simulink model "APP_MyApplication"  (R2018b)
settings: Solver=VariableStepDiscrete  StartTime=0.0  StopTime=10  RelTol=1e-3
PreLoadFcn:
  | if(exist('MBDS_ModelCallback', 'file')), MBDS_ModelCallback('PreLoad'); end;
PostLoadFcn:
  | if(exist('MBDS_ModelCallback', 'file')), MBDS_ModelCallback('PostLoad'); end;
InitFcn:
  | if(exist('MBDS_ModelCallback', 'file')), MBDS_ModelCallback('Init'); end;
StartFcn:
  | if(exist('MBDS_ModelCallback', 'file')), MBDS_ModelCallback('Start'); end;
StopFcn:
  | if(exist('MBDS_ModelCallback', 'file')), MBDS_ModelCallback('Stop'); end;
undefined symbols (not defined in the file): sigbuilder_block, Ts
libraries: KIBES_Signal x499, simulink x8
(part 5 of 10)

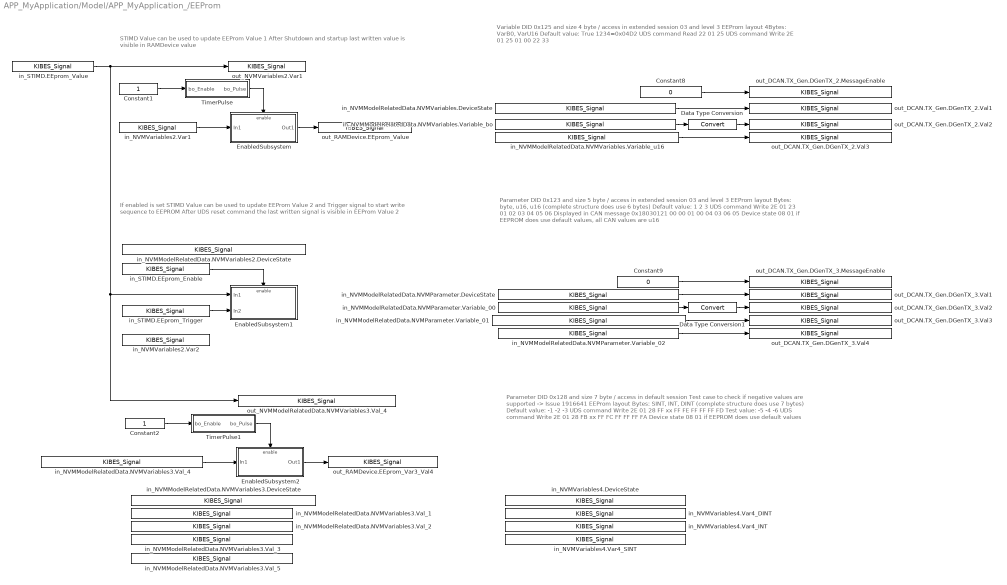
== system APP_MyApplication/Model/APP_MyApplication_/EEProm ==
  note: STIMD Value can be used to update EEProm Value 1
      | After Shutdown and startup last written value is visible in RAMDevice value
  note: Parameter DID 0x123 and size 5 byte / access in extended session 03 and level 3
      | EEProm layout Bytes: byte, u16, u16 (complete structure does use 6 bytes)
      | Default value: 1 2 3
      | UDS command Write 2E 01 23 01 02 03 04 05 06
      | Displayed in CAN message 0x18030121 00 00 01 00 04 03 06 05
      | Device state 08 01 if EEPROM does use default values, all CAN values are u16
  note: Variable DID 0x125 and size 4 byte / access in extended session 03 and level 3
      | EEProm layout 4Bytes: VarB0, VarU16
      | Default value: True 1234=0x04D2
      | UDS command Read 22 01 25
      | UDS command Write 2E 01 25 01 00 22 33
  note: If enabled is set
      | STIMD Value can be used to update EEProm Value 2
      | and Trigger signal to start write sequence to EEPROM
      | After UDS reset command the last written signal is visible in EEProm Value 2
  note: Parameter DID 0x128 and size 7 byte / access in default session
      | Test case to check if negative values are supported -> Issue 1916641
      | EEProm layout Bytes: SINT, INT, DINT (complete structure does use 7 bytes)
      | Default value: -1 -2 -3
      | UDS command Write 2E 01 28 FF xx FF FE FF FF FF FD
      | Test value: -5 -4 -6
      | UDS command Write 2E 01 28 FB xx FF FC FF FF FF FA
      | Device state 08 01 if EEPROM does use default values
  Constant1 : Constant  InitFcn=|  OutDataTypeStr=boolean
      | if(exist('MBDS_BlockCallback', 'file'))
      |    MBDS_BlockCallback('Update', gcb);  
      | end
  Constant2 : Constant  InitFcn=|  OutDataTypeStr=boolean
      | if(exist('MBDS_BlockCallback', 'file'))
      |    MBDS_BlockCallback('Update', gcb);  
      | end
  Constant8 : Constant  InitFcn=|  Value=0  OutDataTypeStr=boolean
      | if(exist('MBDS_BlockCallback', 'file'))
      |    MBDS_BlockCallback('Update', gcb);  
      | end
  Constant9 : Constant  InitFcn=|  Value=0  OutDataTypeStr=boolean
      | if(exist('MBDS_BlockCallback', 'file'))
      |    MBDS_BlockCallback('Update', gcb);  
      | end
  Data Type Conversion : DataTypeConversion  InitFcn=|  SaturateOnIntegerOverflow=on
      | try
      |    MBDS_BlockCallback('Update', gcb);
      | end
      settings: AttributesFormatString=Saturate: %<SaturateOnIntegerOverflow>
  Data Type Conversion1 : DataTypeConversion  InitFcn=|  SaturateOnIntegerOverflow=on
      | try
      |    MBDS_BlockCallback('Update', gcb);
      | end
      settings: AttributesFormatString=Saturate: %<SaturateOnIntegerOverflow>
  EnabledSubsystem : Subsystem
  EnabledSubsystem1 : Subsystem
  EnabledSubsystem2 : Subsystem
  TimerPulse : Subsystem
  TimerPulse1 : Subsystem
  in_NVMModelRelatedData.NVMParameter.DeviceState : KIBES_Signal/KIBES_Signal  MBDS_LibraryBlock=on  DatabaseKey=167  SignalName=NVMModelRelatedData.NVMParameter.DeviceState  SymbolName=NVMModelRelatedData_NVMParameter_DeviceState_000167  DataType=uint16  Init=0  Slope=1  Bias=0  DataSize=1  fpDataType=uint16  BlockIOType=Inport  DeviceType=0
  in_NVMModelRelatedData.NVMParameter.Variable_00 : KIBES_Signal/KIBES_Signal  MBDS_LibraryBlock=on  DatabaseKey=168  SignalName=NVMModelRelatedData.NVMParameter.Variable_00  SymbolName=NVMModelRelatedData_NVMParameter_Variable_00_000168  DataType=uint8  Init=1  Slope=1  Bias=0  DataSize=1  fpDataType=uint8  BlockIOType=Inport  DeviceType=0
  in_NVMModelRelatedData.NVMParameter.Variable_01 : KIBES_Signal/KIBES_Signal  MBDS_LibraryBlock=on  DatabaseKey=169  SignalName=NVMModelRelatedData.NVMParameter.Variable_01  SymbolName=NVMModelRelatedData_NVMParameter_Variable_01_000169  DataType=uint16  Init=0  Slope=1  Bias=0  DataSize=1  fpDataType=uint16  BlockIOType=Inport  DeviceType=0
  in_NVMModelRelatedData.NVMParameter.Variable_02 : KIBES_Signal/KIBES_Signal  MBDS_LibraryBlock=on  DatabaseKey=170  SignalName=NVMModelRelatedData.NVMParameter.Variable_02  SymbolName=NVMModelRelatedData_NVMParameter_Variable_02_000170  DataType=uint16  Init=3  Slope=1  Bias=0  DataSize=1  fpDataType=uint16  BlockIOType=Inport  DeviceType=0
  in_NVMModelRelatedData.NVMVariables.DeviceState : KIBES_Signal/KIBES_Signal  MBDS_LibraryBlock=on  DatabaseKey=160  SignalName=NVMModelRelatedData.NVMVariables.DeviceState  SymbolName=NVMModelRelatedData_NVMVariables_DeviceState_000160  DataType=uint16  Init=0  Slope=1  Bias=0  DataSize=1  fpDataType=uint16  BlockIOType=Inport  DeviceType=0
  in_NVMModelRelatedData.NVMVariables.Variable_bo : KIBES_Signal/KIBES_Signal  MBDS_LibraryBlock=on  DatabaseKey=161  SignalName=NVMModelRelatedData.NVMVariables.Variable_bo  SymbolName=NVMModelRelatedData_NVMVariables_Variable_bo_000161  DataType=boolean  Init=1  Slope=1  Bias=0  DataSize=1  fpDataType=boolean  BlockIOType=Inport  DeviceType=0
  in_NVMModelRelatedData.NVMVariables.Variable_u16 : KIBES_Signal/KIBES_Signal  MBDS_LibraryBlock=on  DatabaseKey=162  SignalName=NVMModelRelatedData.NVMVariables.Variable_u16  SymbolName=NVMModelRelatedData_NVMVariables_Variable_u16_000162  DataType=uint16  Init=1234  Slope=1  Bias=0  DataSize=1  fpDataType=uint16  BlockIOType=Inport  DeviceType=0
  in_NVMModelRelatedData.NVMVariables2.DeviceState : KIBES_Signal/KIBES_Signal  MBDS_LibraryBlock=on  DatabaseKey=439  SignalName=NVMModelRelatedData.NVMVariables2.DeviceState  SymbolName=NVMModelRelatedData_NVMVariables2_DeviceState_000439  DataType=uint16  Init=0  Slope=1  Bias=0  DataSize=1  fpDataType=uint16  BlockIOType=Inport  DeviceType=0
  in_NVMModelRelatedData.NVMVariables3.DeviceState : KIBES_Signal/KIBES_Signal  MBDS_LibraryBlock=on  DatabaseKey=536  SignalName=NVMModelRelatedData.NVMVariables3.DeviceState  SymbolName=NVMModelRelatedData_NVMVariables3_DeviceState_000536  DataType=uint16  Init=0  Slope=1  Bias=0  DataSize=1  fpDataType=uint16  BlockIOType=Inport  DeviceType=0
  in_NVMModelRelatedData.NVMVariables3.Val_1 : KIBES_Signal/KIBES_Signal  MBDS_LibraryBlock=on  DatabaseKey=537  SignalName=NVMModelRelatedData.NVMVariables3.Val_1  SymbolName=NVMModelRelatedData_NVMVariables3_Val_1_000537  DataType=boolean  Init=1  Slope=1  Bias=0  DataSize=1  fpDataType=boolean  BlockIOType=Inport  DeviceType=0
  in_NVMModelRelatedData.NVMVariables3.Val_2 : KIBES_Signal/KIBES_Signal  MBDS_LibraryBlock=on  DatabaseKey=538  SignalName=NVMModelRelatedData.NVMVariables3.Val_2  SymbolName=NVMModelRelatedData_NVMVariables3_Val_2_000538  DataType=uint8  Init=2  Slope=1  Bias=0  DataSize=1  fpDataType=uint8  BlockIOType=Inport  DeviceType=0
  in_NVMModelRelatedData.NVMVariables3.Val_3 : KIBES_Signal/KIBES_Signal  MBDS_LibraryBlock=on  DatabaseKey=539  SignalName=NVMModelRelatedData.NVMVariables3.Val_3  SymbolName=NVMModelRelatedData_NVMVariables3_Val_3_000539  DataType=uint16  Init=3  Slope=1  Bias=0  DataSize=1  fpDataType=uint16  BlockIOType=Inport  DeviceType=0
  in_NVMModelRelatedData.NVMVariables3.Val_4 : KIBES_Signal/KIBES_Signal  MBDS_LibraryBlock=on  DatabaseKey=540  SignalName=NVMModelRelatedData.NVMVariables3.Val_4  SymbolName=NVMModelRelatedData_NVMVariables3_Val_4_000540  DataType=uint32  Init=4  Slope=1  Bias=0  DataSize=1  fpDataType=uint32  BlockIOType=Inport  DeviceType=0
  in_NVMModelRelatedData.NVMVariables3.Val_5 : KIBES_Signal/KIBES_Signal  MBDS_LibraryBlock=on  DatabaseKey=542  SignalName=NVMModelRelatedData.NVMVariables3.Val_5  SymbolName=NVMModelRelatedData_NVMVariables3_Val_5_000542  DataType=uint8  Init=0  Slope=1  Bias=0  DataSize=1  fpDataType=uint8  BlockIOType=Inport  DeviceType=0
  in_NVMVariables2.Var1 : KIBES_Signal/KIBES_Signal  MBDS_LibraryBlock=on  DatabaseKey=438  SignalName=NVMVariables2.Var1  SymbolName=NVMVariables2_Var1_000438  DataType=uint32  Init=0  Slope=1  Bias=0  DataSize=1  fpDataType=uint32  BlockIOType=Inport  DeviceType=0
  in_NVMVariables2.Var2 : KIBES_Signal/KIBES_Signal  MBDS_LibraryBlock=on  DatabaseKey=437  SignalName=NVMVariables2.Var2  SymbolName=NVMVariables2_Var2_000437  DataType=uint32  Init=0  Slope=1  Bias=0  DataSize=1  fpDataType=uint32  BlockIOType=Inport  DeviceType=0
  in_NVMVariables4.DeviceState : KIBES_Signal/KIBES_Signal  MBDS_LibraryBlock=on  DatabaseKey=607  SignalName=NVMVariables4.DeviceState  SymbolName=NVMVariables4_DeviceState_000607  DataType=uint16  Init=0  Slope=1  Bias=0  DataSize=1  fpDataType=uint16  BlockIOType=Inport  DeviceType=0
  in_NVMVariables4.Var4_DINT : KIBES_Signal/KIBES_Signal  MBDS_LibraryBlock=on  DatabaseKey=605  SignalName=NVMVariables4.Var4_DINT  SymbolName=NVMVariables4_Var4_DINT_000605  DataType=int32  Init=0  Slope=1  Bias=0  DataSize=1  fpDataType=int32  BlockIOType=Inport  DeviceType=0
  in_NVMVariables4.Var4_INT : KIBES_Signal/KIBES_Signal  MBDS_LibraryBlock=on  DatabaseKey=604  SignalName=NVMVariables4.Var4_INT  SymbolName=NVMVariables4_Var4_INT_000604  DataType=int16  Init=0  Slope=1  Bias=0  DataSize=1  fpDataType=int16  BlockIOType=Inport  DeviceType=0
  in_NVMVariables4.Var4_SINT : KIBES_Signal/KIBES_Signal  MBDS_LibraryBlock=on  DatabaseKey=606  SignalName=NVMVariables4.Var4_SINT  SymbolName=NVMVariables4_Var4_SINT_000606  DataType=int8  Init=0  Slope=1  Bias=0  DataSize=1  fpDataType=int8  BlockIOType=Inport  DeviceType=0
  in_STIMD.EEprom_Enable : KIBES_Signal/KIBES_Signal  MBDS_LibraryBlock=on  DatabaseKey=433  SignalName=STIMD.EEprom_Enable  SymbolName=STIMD_EEprom_Enable_000433  DataType=boolean  Init=0  Slope=1  Bias=0  DataSize=1  fpDataType=boolean  BlockIOType=Inport  DeviceType=2
  in_STIMD.EEprom_Trigger : KIBES_Signal/KIBES_Signal  MBDS_LibraryBlock=on  DatabaseKey=434  SignalName=STIMD.EEprom_Trigger  SymbolName=STIMD_EEprom_Trigger_000434  DataType=boolean  Init=0  Slope=1  Bias=0  DataSize=1  fpDataType=boolean  BlockIOType=Inport  DeviceType=2
  in_STIMD.EEprom_Value : KIBES_Signal/KIBES_Signal  MBDS_LibraryBlock=on  DatabaseKey=435  SignalName=STIMD.EEprom_Value  SymbolName=STIMD_EEprom_Value_000435  DataType=uint32  Init=0  Slope=1  Bias=0  DataSize=1  fpDataType=uint32  BlockIOType=Inport  DeviceType=2
  out_DCAN.TX_Gen.DGenTX_2.MessageEnable : KIBES_Signal/KIBES_Signal  MBDS_LibraryBlock=on  DatabaseKey=163  SignalName=DCAN.TX_Gen.DGenTX_2.MessageEnable  SymbolName=DCAN_TX_Gen_DGenTX_2_MessageEnable_000163  DataType=boolean  Init=0  Slope=1  Bias=0  DataSize=1  fpDataType=boolean  BlockIOType=Outport  DeviceType=0
  out_DCAN.TX_Gen.DGenTX_2.Val1 : KIBES_Signal/KIBES_Signal  MBDS_LibraryBlock=on  DatabaseKey=164  SignalName=DCAN.TX_Gen.DGenTX_2.Val1  SymbolName=DCAN_TX_Gen_DGenTX_2_Val1_000164  DataType=uint16  Init=0  Slope=1  Bias=0  DataSize=1  fpDataType=uint16  BlockIOType=Outport  DeviceType=0
  out_DCAN.TX_Gen.DGenTX_2.Val2 : KIBES_Signal/KIBES_Signal  MBDS_LibraryBlock=on  DatabaseKey=165  SignalName=DCAN.TX_Gen.DGenTX_2.Val2  SymbolName=DCAN_TX_Gen_DGenTX_2_Val2_000165  DataType=uint16  Init=0  Slope=1  Bias=0  DataSize=1  fpDataType=uint16  BlockIOType=Outport  DeviceType=0
  out_DCAN.TX_Gen.DGenTX_2.Val3 : KIBES_Signal/KIBES_Signal  MBDS_LibraryBlock=on  DatabaseKey=166  SignalName=DCAN.TX_Gen.DGenTX_2.Val3  SymbolName=DCAN_TX_Gen_DGenTX_2_Val3_000166  DataType=uint16  Init=0  Slope=1  Bias=0  DataSize=1  fpDataType=uint16  BlockIOType=Outport  DeviceType=0
  out_DCAN.TX_Gen.DGenTX_3.MessageEnable : KIBES_Signal/KIBES_Signal  MBDS_LibraryBlock=on  DatabaseKey=171  SignalName=DCAN.TX_Gen.DGenTX_3.MessageEnable  SymbolName=DCAN_TX_Gen_DGenTX_3_MessageEnable_000171  DataType=boolean  Init=0  Slope=1  Bias=0  DataSize=1  fpDataType=boolean  BlockIOType=Outport  DeviceType=0
  out_DCAN.TX_Gen.DGenTX_3.Val1 : KIBES_Signal/KIBES_Signal  MBDS_LibraryBlock=on  DatabaseKey=172  SignalName=DCAN.TX_Gen.DGenTX_3.Val1  SymbolName=DCAN_TX_Gen_DGenTX_3_Val1_000172  DataType=uint16  Init=0  Slope=1  Bias=0  DataSize=1  fpDataType=uint16  BlockIOType=Outport  DeviceType=0
  out_DCAN.TX_Gen.DGenTX_3.Val2 : KIBES_Signal/KIBES_Signal  MBDS_LibraryBlock=on  DatabaseKey=173  SignalName=DCAN.TX_Gen.DGenTX_3.Val2  SymbolName=DCAN_TX_Gen_DGenTX_3_Val2_000173  DataType=uint16  Init=0  Slope=1  Bias=0  DataSize=1  fpDataType=uint16  BlockIOType=Outport  DeviceType=0
  out_DCAN.TX_Gen.DGenTX_3.Val3 : KIBES_Signal/KIBES_Signal  MBDS_LibraryBlock=on  DatabaseKey=174  SignalName=DCAN.TX_Gen.DGenTX_3.Val3  SymbolName=DCAN_TX_Gen_DGenTX_3_Val3_000174  DataType=uint16  Init=0  Slope=1  Bias=0  DataSize=1  fpDataType=uint16  BlockIOType=Outport  DeviceType=0
  out_DCAN.TX_Gen.DGenTX_3.Val4 : KIBES_Signal/KIBES_Signal  MBDS_LibraryBlock=on  DatabaseKey=175  SignalName=DCAN.TX_Gen.DGenTX_3.Val4  SymbolName=DCAN_TX_Gen_DGenTX_3_Val4_000175  DataType=uint16  Init=0  Slope=1  Bias=0  DataSize=1  fpDataType=uint16  BlockIOType=Outport  DeviceType=0
  out_NVMModelRelatedData.NVMVariables3.Val_4 : KIBES_Signal/KIBES_Signal  MBDS_LibraryBlock=on  DatabaseKey=540  SignalName=NVMModelRelatedData.NVMVariables3.Val_4  SymbolName=NVMModelRelatedData_NVMVariables3_Val_4_000540  DataType=uint32  Init=4  Slope=1  Bias=0  DataSize=1  fpDataType=uint32  BlockIOType=Outport  DeviceType=0
  out_NVMVariables2.Var1 : KIBES_Signal/KIBES_Signal  MBDS_LibraryBlock=on  DatabaseKey=438  SignalName=NVMVariables2.Var1  SymbolName=NVMVariables2_Var1_000438  DataType=uint32  Init=0  Slope=1  Bias=0  DataSize=1  fpDataType=uint32  BlockIOType=Outport  DeviceType=0
  out_RAMDevice.EEprom_Value : KIBES_Signal/KIBES_Signal  MBDS_LibraryBlock=on  DatabaseKey=436  SignalName=RAMDevice.EEprom_Value  SymbolName=RAMDevice_EEprom_Value_000436  DataType=uint32  Init=0  Slope=1  Bias=0  DataSize=1  fpDataType=uint32  BlockIOType=Outport  DeviceType=0
  out_RAMDevice.EEprom_Var3_Val4 : KIBES_Signal/KIBES_Signal  MBDS_LibraryBlock=on  DatabaseKey=541  SignalName=RAMDevice.EEprom_Var3_Val4  SymbolName=RAMDevice_EEprom_Var3_Val4_000541  DataType=uint32  Init=0  Slope=1  Bias=0  DataSize=1  fpDataType=uint32  BlockIOType=Outport  DeviceType=0
  wires:
  in_NVMModelRelatedData.NVMVariables.Variable_u16/1 -> out_DCAN.TX_Gen.DGenTX_2.Val3/1
  in_NVMModelRelatedData.NVMParameter.Variable_01/1 -> out_DCAN.TX_Gen.DGenTX_3.Val3/1
  in_NVMModelRelatedData.NVMParameter.Variable_02/1 -> out_DCAN.TX_Gen.DGenTX_3.Val4/1
  Data Type Conversion1/1 -> out_DCAN.TX_Gen.DGenTX_3.Val2/1
  in_NVMModelRelatedData.NVMVariables.Variable_bo/1 -> Data Type Conversion/1
  in_NVMModelRelatedData.NVMParameter.DeviceState/1 -> out_DCAN.TX_Gen.DGenTX_3.Val1/1
  Data Type Conversion/1 -> out_DCAN.TX_Gen.DGenTX_2.Val2/1
  in_NVMModelRelatedData.NVMParameter.Variable_00/1 -> Data Type Conversion1/1
  in_NVMModelRelatedData.NVMVariables.DeviceState/1 -> out_DCAN.TX_Gen.DGenTX_2.Val1/1
  Constant8/1 -> out_DCAN.TX_Gen.DGenTX_2.MessageEnable/1
  Constant9/1 -> out_DCAN.TX_Gen.DGenTX_3.MessageEnable/1
  Constant1/1 -> TimerPulse/1(bo_Enable)
  TimerPulse/1(bo_Pulse) -> EnabledSubsystem/Enable
  in_NVMVariables2.Var1/1 -> EnabledSubsystem/1(In1)
  EnabledSubsystem/1(Out1) -> out_RAMDevice.EEprom_Value/1
  in_STIMD.EEprom_Enable/1 -> EnabledSubsystem1/Enable
  in_STIMD.EEprom_Trigger/1 -> EnabledSubsystem1/2(In2)
  in_NVMModelRelatedData.NVMVariables3.Val_4/1 -> EnabledSubsystem2/1(In1)
  in_STIMD.EEprom_Value/1 -> out_NVMVariables2.Var1/1, out_NVMModelRelatedData.NVMVariables3.Val_4/1, EnabledSubsystem1/1("In1 ")
  EnabledSubsystem2/1(Out1) -> out_RAMDevice.EEprom_Var3_Val4/1
  Constant2/1 -> TimerPulse1/1(bo_Enable)
  TimerPulse1/1(bo_Pulse) -> EnabledSubsystem2/Enable

== system APP_MyApplication/Model/APP_MyApplication_/FMS-CAN(5) DM1RX ==
  note: 18010521
  note: DM1RX
  Constant1 : Constant  InitFcn=|  Value=55  OutDataTypeStr=uint8
      | if(exist('MBDS_BlockCallback', 'file'))
      |    MBDS_BlockCallback('Update', gcb);  
      | end
  Constant2 : Constant  InitFcn=|  OutDataTypeStr=boolean
      | if(exist('MBDS_BlockCallback', 'file'))
      |    MBDS_BlockCallback('Update', gcb);  
      | end
  in_FMSCAN.BusActivityState : KIBES_Signal/KIBES_Signal  MBDS_LibraryBlock=on  DatabaseKey=429  SignalName=FMSCAN.BusActivityState  SymbolName=FMSCAN_BusActivityState_000429  DataType=boolean  Init=0  Slope=1  Bias=0  DataSize=1  fpDataType=boolean  BlockIOType=Inport  DeviceType=0
  in_FMSCAN.GenericDM1RxSA11.ActiveDTC : KIBES_Signal/KIBES_Signal  MBDS_LibraryBlock=on  DatabaseKey=443  SignalName=FMSCAN.GenericDM1RxSA11.ActiveDTC  SymbolName=FMSCAN_GenericDM1RxSA11_ActiveDTC_000443  DataType=boolean  Init=0  Slope=1  Bias=0  DataSize=1  fpDataType=boolean  BlockIOType=Inport  DeviceType=0
  in_FMSCAN.GenericDM1RxSA11.AmberWarningLamp : KIBES_Signal/KIBES_Signal  MBDS_LibraryBlock=on  DatabaseKey=444  SignalName=FMSCAN.GenericDM1RxSA11.AmberWarningLamp  SymbolName=FMSCAN_GenericDM1RxSA11_AmberWarningLamp_000444  DataType=boolean  Init=0  Slope=1  Bias=0  DataSize=1  fpDataType=boolean  BlockIOType=Inport  DeviceType=0
  in_FMSCAN.GenericDM1RxSA11.AmberWarningLampFlash : KIBES_Signal/KIBES_Signal  MBDS_LibraryBlock=on  DatabaseKey=445  SignalName=FMSCAN.GenericDM1RxSA11.AmberWarningLampFlash  SymbolName=FMSCAN_GenericDM1RxSA11_AmberWarningLampFlash_000445  DataType=uint8  Init=0  Slope=1  Bias=0  DataSize=1  fpDataType=uint8  BlockIOType=Inport  DeviceType=0
  in_FMSCAN.GenericDM1RxSA11.MessageState : KIBES_Signal/KIBES_Signal  MBDS_LibraryBlock=on  DatabaseKey=447  SignalName=FMSCAN.GenericDM1RxSA11.MessageState  SymbolName=FMSCAN_GenericDM1RxSA11_MessageState_000447  DataType=uint16  Init=0  Slope=1  Bias=0  DataSize=1  fpDataType=uint16  BlockIOType=Inport  DeviceType=0
  in_FMSCAN.GenericDM1RxSA11.UndefinedActiveDtc : KIBES_Signal/KIBES_Signal  MBDS_LibraryBlock=on  DatabaseKey=448  SignalName=FMSCAN.GenericDM1RxSA11.UndefinedActiveDtc  SymbolName=FMSCAN_GenericDM1RxSA11_UndefinedActiveDtc_000448  DataType=boolean  Init=0  Slope=1  Bias=0  DataSize=1  fpDataType=boolean  BlockIOType=Inport  DeviceType=0
  in_FMSCAN.TX_GEN.FMSGenTX_1.MessageState : KIBES_Signal/KIBES_Signal  MBDS_LibraryBlock=on  DatabaseKey=298  SignalName=FMSCAN.TX_GEN.FMSGenTX_1.MessageState  SymbolName=FMSCAN_TX_GEN_FMSGenTX_1_MessageState_000298  DataType=uint16  Init=0  Slope=1  Bias=0  DataSize=1  fpDataType=uint16  BlockIOType=Inport  DeviceType=0
  in_STIMD.FmsCanEnable : KIBES_Signal/KIBES_Signal  MBDS_LibraryBlock=on  DatabaseKey=441  SignalName=STIMD.FmsCanEnable  SymbolName=STIMD_FmsCanEnable_000441  DataType=boolean  Init=0  Slope=1  Bias=0  DataSize=1  fpDataType=boolean  BlockIOType=Inport  DeviceType=2
  out_FMSCAN.GenericDM1RxSA11.MessageEnable : KIBES_Signal/KIBES_Signal  MBDS_LibraryBlock=on  DatabaseKey=446  SignalName=FMSCAN.GenericDM1RxSA11.MessageEnable  SymbolName=FMSCAN_GenericDM1RxSA11_MessageEnable_000446  DataType=boolean  Init=0  Slope=1  Bias=0  DataSize=1  fpDataType=boolean  BlockIOType=Outport  DeviceType=0
  out_FMSCAN.TX_GEN.FMSGenTX_1.MessageEnable : KIBES_Signal/KIBES_Signal  MBDS_LibraryBlock=on  DatabaseKey=297  SignalName=FMSCAN.TX_GEN.FMSGenTX_1.MessageEnable  SymbolName=FMSCAN_TX_GEN_FMSGenTX_1_MessageEnable_000297  DataType=boolean  Init=0  Slope=1  Bias=0  DataSize=1  fpDataType=boolean  BlockIOType=Outport  DeviceType=0
  out_FMSCAN.TX_GEN.FMSGenTX_1.Val_1 : KIBES_Signal/KIBES_Signal  MBDS_LibraryBlock=on  DatabaseKey=299  SignalName=FMSCAN.TX_GEN.FMSGenTX_1.Val_1  SymbolName=FMSCAN_TX_GEN_FMSGenTX_1_Val_1_000299  DataType=uint8  Init=0  Slope=1  Bias=0  DataSize=1  fpDataType=uint8  BlockIOType=Outport  DeviceType=0
  wires:
  in_STIMD.FmsCanEnable/1 -> out_FMSCAN.TX_GEN.FMSGenTX_1.MessageEnable/1
  Constant1/1 -> out_FMSCAN.TX_GEN.FMSGenTX_1.Val_1/1
  Constant2/1 -> out_FMSCAN.GenericDM1RxSA11.MessageEnable/1

== system APP_MyApplication/Model/APP_MyApplication_/H-CAN(7) 500kBaud ==
  Constant1 : Constant  InitFcn=|  OutDataTypeStr=uint8
      | if(exist('MBDS_BlockCallback', 'file'))
      |    MBDS_BlockCallback('Update', gcb);  
      | end
  Constant2 : Constant  InitFcn=|  Value=2  OutDataTypeStr=uint8
      | if(exist('MBDS_BlockCallback', 'file'))
      |    MBDS_BlockCallback('Update', gcb);  
      | end
  Constant7 : Constant  InitFcn=|  OutDataTypeStr=boolean
      | if(exist('MBDS_BlockCallback', 'file'))
      |    MBDS_BlockCallback('Update', gcb);  
      | end
  in_HCAN.TX_GEN.HGenTX_1.MessageState : KIBES_Signal/KIBES_Signal  MBDS_LibraryBlock=on  DatabaseKey=265  SignalName=HCAN.TX_GEN.HGenTX_1.MessageState  SymbolName=HCAN_TX_GEN_HGenTX_1_MessageState_000265  DataType=uint16  Init=0  Slope=1  Bias=0  DataSize=1  fpDataType=uint16  BlockIOType=Inport  DeviceType=0
  out_HCAN.TX_GEN.HGenTX_1.MessageEnable : KIBES_Signal/KIBES_Signal  MBDS_LibraryBlock=on  DatabaseKey=264  SignalName=HCAN.TX_GEN.HGenTX_1.MessageEnable  SymbolName=HCAN_TX_GEN_HGenTX_1_MessageEnable_000264  DataType=boolean  Init=0  Slope=1  Bias=0  DataSize=1  fpDataType=boolean  BlockIOType=Outport  DeviceType=0
  out_HCAN.TX_GEN.HGenTX_1.Val_1 : KIBES_Signal/KIBES_Signal  MBDS_LibraryBlock=on  DatabaseKey=266  SignalName=HCAN.TX_GEN.HGenTX_1.Val_1  SymbolName=HCAN_TX_GEN_HGenTX_1_Val_1_000266  DataType=uint8  Init=0  Slope=1  Bias=0  DataSize=1  fpDataType=uint8  BlockIOType=Outport  DeviceType=0
  out_HCAN.TX_GEN.HGenTX_1.Val_2 : KIBES_Signal/KIBES_Signal  MBDS_LibraryBlock=on  DatabaseKey=267  SignalName=HCAN.TX_GEN.HGenTX_1.Val_2  SymbolName=HCAN_TX_GEN_HGenTX_1_Val_2_000267  DataType=uint8  Init=0  Slope=1  Bias=0  DataSize=1  fpDataType=uint8  BlockIOType=Outport  DeviceType=0
  wires:
  Constant7/1 -> out_HCAN.TX_GEN.HGenTX_1.MessageEnable/1
  Constant1/1 -> out_HCAN.TX_GEN.HGenTX_1.Val_1/1
  Constant2/1 -> out_HCAN.TX_GEN.HGenTX_1.Val_2/1

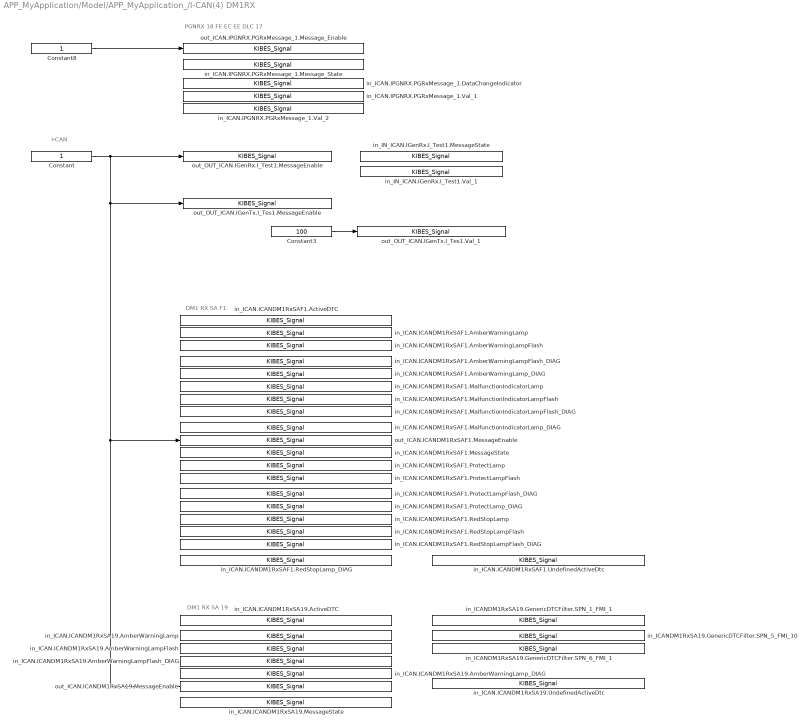
== system APP_MyApplication/Model/APP_MyApplication_/I-CAN(4) DM1RX ==
  note: PGNRX 18 FE EC EE DLC 17
  note: DM1 RX SA F1
  note: I-CAN
  note: DM1 RX SA 19
  Constant : Constant  InitFcn=|  OutDataTypeStr=boolean
      | if(exist('MBDS_BlockCallback', 'file'))
      |    MBDS_BlockCallback('Update', gcb);  
      | end
  Constant3 : Constant  InitFcn=|  Value=100  OutDataTypeStr=uint8
      | if(exist('MBDS_BlockCallback', 'file'))
      |    MBDS_BlockCallback('Update', gcb);  
      | end
  Constant8 : Constant  InitFcn=|  OutDataTypeStr=boolean
      | if(exist('MBDS_BlockCallback', 'file'))
      |    MBDS_BlockCallback('Update', gcb);  
      | end
  in_ICAN.ICANDM1RxSA19.ActiveDTC : KIBES_Signal/KIBES_Signal  MBDS_LibraryBlock=on  DatabaseKey=149  SignalName=ICAN.ICANDM1RxSA19.ActiveDTC  SymbolName=ICAN_ICANDM1RxSA19_ActiveDTC_000149  DataType=boolean  Init=0  Slope=1  Bias=0  DataSize=1  fpDataType=boolean  BlockIOType=Inport  DeviceType=0
  in_ICAN.ICANDM1RxSA19.AmberWarningLamp : KIBES_Signal/KIBES_Signal  MBDS_LibraryBlock=on  DatabaseKey=150  SignalName=ICAN.ICANDM1RxSA19.AmberWarningLamp  SymbolName=ICAN_ICANDM1RxSA19_AmberWarningLamp_000150  DataType=boolean  Init=0  Slope=1  Bias=0  DataSize=1  fpDataType=boolean  BlockIOType=Inport  DeviceType=0
  in_ICAN.ICANDM1RxSA19.AmberWarningLampFlash : KIBES_Signal/KIBES_Signal  MBDS_LibraryBlock=on  DatabaseKey=151  SignalName=ICAN.ICANDM1RxSA19.AmberWarningLampFlash  SymbolName=ICAN_ICANDM1RxSA19_AmberWarningLampFlash_000151  DataType=uint8  Init=0  Slope=1  Bias=0  DataSize=1  fpDataType=uint8  BlockIOType=Inport  DeviceType=0
  in_ICAN.ICANDM1RxSA19.AmberWarningLampFlash_DIAG : KIBES_Signal/KIBES_Signal  MBDS_LibraryBlock=on  DatabaseKey=152  SignalName=ICAN.ICANDM1RxSA19.AmberWarningLampFlash_DIAG  SymbolName=ICAN_ICANDM1RxSA19_AmberWarningLampFlash_DIAG_000152  DataType=uint16  Init=1  Slope=1  Bias=0  DataSize=1  fpDataType=uint16  BlockIOType=Inport  DeviceType=0
  in_ICAN.ICANDM1RxSA19.AmberWarningLamp_DIAG : KIBES_Signal/KIBES_Signal  MBDS_LibraryBlock=on  DatabaseKey=153  SignalName=ICAN.ICANDM1RxSA19.AmberWarningLamp_DIAG  SymbolName=ICAN_ICANDM1RxSA19_AmberWarningLamp_DIAG_000153  DataType=uint16  Init=1  Slope=1  Bias=0  DataSize=1  fpDataType=uint16  BlockIOType=Inport  DeviceType=0
  in_ICAN.ICANDM1RxSA19.MessageState : KIBES_Signal/KIBES_Signal  MBDS_LibraryBlock=on  DatabaseKey=155  SignalName=ICAN.ICANDM1RxSA19.MessageState  SymbolName=ICAN_ICANDM1RxSA19_MessageState_000155  DataType=uint16  Init=0  Slope=1  Bias=0  DataSize=1  fpDataType=uint16  BlockIOType=Inport  DeviceType=0
  in_ICAN.ICANDM1RxSA19.UndefinedActiveDtc : KIBES_Signal/KIBES_Signal  MBDS_LibraryBlock=on  DatabaseKey=401  SignalName=ICAN.ICANDM1RxSA19.UndefinedActiveDtc  SymbolName=ICAN_ICANDM1RxSA19_UndefinedActiveDtc_000401  DataType=boolean  Init=0  Slope=1  Bias=0  DataSize=1  fpDataType=boolean  BlockIOType=Inport  DeviceType=0
  in_ICAN.ICANDM1RxSAF1.ActiveDTC : KIBES_Signal/KIBES_Signal  MBDS_LibraryBlock=on  DatabaseKey=129  SignalName=ICAN.ICANDM1RxSAF1.ActiveDTC  SymbolName=ICAN_ICANDM1RxSAF1_ActiveDTC_000129  DataType=boolean  Init=0  Slope=1  Bias=0  DataSize=1  fpDataType=boolean  BlockIOType=Inport  DeviceType=0
  in_ICAN.ICANDM1RxSAF1.AmberWarningLamp : KIBES_Signal/KIBES_Signal  MBDS_LibraryBlock=on  DatabaseKey=130  SignalName=ICAN.ICANDM1RxSAF1.AmberWarningLamp  SymbolName=ICAN_ICANDM1RxSAF1_AmberWarningLamp_000130  DataType=boolean  Init=0  Slope=1  Bias=0  DataSize=1  fpDataType=boolean  BlockIOType=Inport  DeviceType=0
  in_ICAN.ICANDM1RxSAF1.AmberWarningLampFlash : KIBES_Signal/KIBES_Signal  MBDS_LibraryBlock=on  DatabaseKey=131  SignalName=ICAN.ICANDM1RxSAF1.AmberWarningLampFlash  SymbolName=ICAN_ICANDM1RxSAF1_AmberWarningLampFlash_000131  DataType=uint8  Init=0  Slope=1  Bias=0  DataSize=1  fpDataType=uint8  BlockIOType=Inport  DeviceType=0
  in_ICAN.ICANDM1RxSAF1.AmberWarningLampFlash_DIAG : KIBES_Signal/KIBES_Signal  MBDS_LibraryBlock=on  DatabaseKey=132  SignalName=ICAN.ICANDM1RxSAF1.AmberWarningLampFlash_DIAG  SymbolName=ICAN_ICANDM1RxSAF1_AmberWarningLampFlash_DIAG_000132  DataType=uint16  Init=1  Slope=1  Bias=0  DataSize=1  fpDataType=uint16  BlockIOType=Inport  DeviceType=0
  in_ICAN.ICANDM1RxSAF1.AmberWarningLamp_DIAG : KIBES_Signal/KIBES_Signal  MBDS_LibraryBlock=on  DatabaseKey=133  SignalName=ICAN.ICANDM1RxSAF1.AmberWarningLamp_DIAG  SymbolName=ICAN_ICANDM1RxSAF1_AmberWarningLamp_DIAG_000133  DataType=uint16  Init=1  Slope=1  Bias=0  DataSize=1  fpDataType=uint16  BlockIOType=Inport  DeviceType=0
  in_ICAN.ICANDM1RxSAF1.MalfunctionIndicatorLamp : KIBES_Signal/KIBES_Signal  MBDS_LibraryBlock=on  DatabaseKey=134  SignalName=ICAN.ICANDM1RxSAF1.MalfunctionIndicatorLamp  SymbolName=ICAN_ICANDM1RxSAF1_MalfunctionIndicatorLamp_000134  DataType=boolean  Init=0  Slope=1  Bias=0  DataSize=1  fpDataType=boolean  BlockIOType=Inport  DeviceType=0
  in_ICAN.ICANDM1RxSAF1.MalfunctionIndicatorLampFlash : KIBES_Signal/KIBES_Signal  MBDS_LibraryBlock=on  DatabaseKey=135  SignalName=ICAN.ICANDM1RxSAF1.MalfunctionIndicatorLampFlash  SymbolName=ICAN_ICANDM1RxSAF1_MalfunctionIndicatorLampFlash_000135  DataType=uint8  Init=0  Slope=1  Bias=0  DataSize=1  fpDataType=uint8  BlockIOType=Inport  DeviceType=0
  in_ICAN.ICANDM1RxSAF1.MalfunctionIndicatorLampFlash_DIAG : KIBES_Signal/KIBES_Signal  MBDS_LibraryBlock=on  DatabaseKey=136  SignalName=ICAN.ICANDM1RxSAF1.MalfunctionIndicatorLampFlash_DIAG  SymbolName=ICAN_ICANDM1RxSAF1_MalfunctionIndicatorLampFlash_DIAG_000136  DataType=uint16  Init=1  Slope=1  Bias=0  DataSize=1  fpDataType=uint16  BlockIOType=Inport  DeviceType=0
  in_ICAN.ICANDM1RxSAF1.MalfunctionIndicatorLamp_DIAG : KIBES_Signal/KIBES_Signal  MBDS_LibraryBlock=on  DatabaseKey=137  SignalName=ICAN.ICANDM1RxSAF1.MalfunctionIndicatorLamp_DIAG  SymbolName=ICAN_ICANDM1RxSAF1_MalfunctionIndicatorLamp_DIAG_000137  DataType=uint16  Init=1  Slope=1  Bias=0  DataSize=1  fpDataType=uint16  BlockIOType=Inport  DeviceType=0
  in_ICAN.ICANDM1RxSAF1.MessageState : KIBES_Signal/KIBES_Signal  MBDS_LibraryBlock=on  DatabaseKey=139  SignalName=ICAN.ICANDM1RxSAF1.MessageState  SymbolName=ICAN_ICANDM1RxSAF1_MessageState_000139  DataType=uint16  Init=0  Slope=1  Bias=0  DataSize=1  fpDataType=uint16  BlockIOType=Inport  DeviceType=0
  in_ICAN.ICANDM1RxSAF1.ProtectLamp : KIBES_Signal/KIBES_Signal  MBDS_LibraryBlock=on  DatabaseKey=140  SignalName=ICAN.ICANDM1RxSAF1.ProtectLamp  SymbolName=ICAN_ICANDM1RxSAF1_ProtectLamp_000140  DataType=boolean  Init=0  Slope=1  Bias=0  DataSize=1  fpDataType=boolean  BlockIOType=Inport  DeviceType=0
  in_ICAN.ICANDM1RxSAF1.ProtectLampFlash : KIBES_Signal/KIBES_Signal  MBDS_LibraryBlock=on  DatabaseKey=141  SignalName=ICAN.ICANDM1RxSAF1.ProtectLampFlash  SymbolName=ICAN_ICANDM1RxSAF1_ProtectLampFlash_000141  DataType=uint8  Init=0  Slope=1  Bias=0  DataSize=1  fpDataType=uint8  BlockIOType=Inport  DeviceType=0
  in_ICAN.ICANDM1RxSAF1.ProtectLampFlash_DIAG : KIBES_Signal/KIBES_Signal  MBDS_LibraryBlock=on  DatabaseKey=142  SignalName=ICAN.ICANDM1RxSAF1.ProtectLampFlash_DIAG  SymbolName=ICAN_ICANDM1RxSAF1_ProtectLampFlash_DIAG_000142  DataType=uint16  Init=1  Slope=1  Bias=0  DataSize=1  fpDataType=uint16  BlockIOType=Inport  DeviceType=0
  in_ICAN.ICANDM1RxSAF1.ProtectLamp_DIAG : KIBES_Signal/KIBES_Signal  MBDS_LibraryBlock=on  DatabaseKey=143  SignalName=ICAN.ICANDM1RxSAF1.ProtectLamp_DIAG  SymbolName=ICAN_ICANDM1RxSAF1_ProtectLamp_DIAG_000143  DataType=uint16  Init=1  Slope=1  Bias=0  DataSize=1  fpDataType=uint16  BlockIOType=Inport  DeviceType=0
  in_ICAN.ICANDM1RxSAF1.RedStopLamp : KIBES_Signal/KIBES_Signal  MBDS_LibraryBlock=on  DatabaseKey=144  SignalName=ICAN.ICANDM1RxSAF1.RedStopLamp  SymbolName=ICAN_ICANDM1RxSAF1_RedStopLamp_000144  DataType=boolean  Init=0  Slope=1  Bias=0  DataSize=1  fpDataType=boolean  BlockIOType=Inport  DeviceType=0
  in_ICAN.ICANDM1RxSAF1.RedStopLampFlash : KIBES_Signal/KIBES_Signal  MBDS_LibraryBlock=on  DatabaseKey=145  SignalName=ICAN.ICANDM1RxSAF1.RedStopLampFlash  SymbolName=ICAN_ICANDM1RxSAF1_RedStopLampFlash_000145  DataType=uint8  Init=0  Slope=1  Bias=0  DataSize=1  fpDataType=uint8  BlockIOType=Inport  DeviceType=0
  in_ICAN.ICANDM1RxSAF1.RedStopLampFlash_DIAG : KIBES_Signal/KIBES_Signal  MBDS_LibraryBlock=on  DatabaseKey=146  SignalName=ICAN.ICANDM1RxSAF1.RedStopLampFlash_DIAG  SymbolName=ICAN_ICANDM1RxSAF1_RedStopLampFlash_DIAG_000146  DataType=uint16  Init=1  Slope=1  Bias=0  DataSize=1  fpDataType=uint16  BlockIOType=Inport  DeviceType=0
  in_ICAN.ICANDM1RxSAF1.RedStopLamp_DIAG : KIBES_Signal/KIBES_Signal  MBDS_LibraryBlock=on  DatabaseKey=147  SignalName=ICAN.ICANDM1RxSAF1.RedStopLamp_DIAG  SymbolName=ICAN_ICANDM1RxSAF1_RedStopLamp_DIAG_000147  DataType=uint16  Init=1  Slope=1  Bias=0  DataSize=1  fpDataType=uint16  BlockIOType=Inport  DeviceType=0
  in_ICAN.ICANDM1RxSAF1.UndefinedActiveDtc : KIBES_Signal/KIBES_Signal  MBDS_LibraryBlock=on  DatabaseKey=402  SignalName=ICAN.ICANDM1RxSAF1.UndefinedActiveDtc  SymbolName=ICAN_ICANDM1RxSAF1_UndefinedActiveDtc_000402  DataType=boolean  Init=0  Slope=1  Bias=0  DataSize=1  fpDataType=boolean  BlockIOType=Inport  DeviceType=0
  in_ICAN.IPGNRX.PGRxMessage_1.DataChangeIndicator : KIBES_Signal/KIBES_Signal  MBDS_LibraryBlock=on  DatabaseKey=451  SignalName=ICAN.IPGNRX.PGRxMessage_1.DataChangeIndicator  SymbolName=ICAN_IPGNRX_PGRxMessage_1_DataChangeIndicator_000451  DataType=boolean  Init=0  Slope=1  Bias=0  DataSize=1  fpDataType=boolean  BlockIOType=Inport  DeviceType=0
  in_ICAN.IPGNRX.PGRxMessage_1.Message_State : KIBES_Signal/KIBES_Signal  MBDS_LibraryBlock=on  DatabaseKey=453  SignalName=ICAN.IPGNRX.PGRxMessage_1.Message_State  SymbolName=ICAN_IPGNRX_PGRxMessage_1_Message_State_000453  DataType=uint16  Init=0  Slope=1  Bias=0  DataSize=1  fpDataType=uint16  BlockIOType=Inport  DeviceType=0
  in_ICAN.IPGNRX.PGRxMessage_1.Val_1 : KIBES_Signal/KIBES_Signal  MBDS_LibraryBlock=on  DatabaseKey=454  SignalName=ICAN.IPGNRX.PGRxMessage_1.Val_1  SymbolName=ICAN_IPGNRX_PGRxMessage_1_Val_1_000454  DataType=uint32  Init=0  Slope=1  Bias=0  DataSize=1  fpDataType=uint32  BlockIOType=Inport  DeviceType=0
  in_ICAN.IPGNRX.PGRxMessage_1.Val_2 : KIBES_Signal/KIBES_Signal  MBDS_LibraryBlock=on  DatabaseKey=455  SignalName=ICAN.IPGNRX.PGRxMessage_1.Val_2  SymbolName=ICAN_IPGNRX_PGRxMessage_1_Val_2_000455  DataType=uint32  Init=0  Slope=1  Bias=0  DataSize=1  fpDataType=uint32  BlockIOType=Inport  DeviceType=0
  in_ICANDM1RxSA19.GenericDTCFilter.SPN_1_FMI_1 : KIBES_Signal/KIBES_Signal  MBDS_LibraryBlock=on  DatabaseKey=157  SignalName=ICANDM1RxSA19.GenericDTCFilter.SPN_1_FMI_1  SymbolName=ICANDM1RxSA19_GenericDTCFilter_SPN_1_FMI_1_000157  DataType=boolean  Init=0  Slope=1  Bias=0  DataSize=1  fpDataType=boolean  BlockIOType=Inport  DeviceType=0
  in_ICANDM1RxSA19.GenericDTCFilter.SPN_5_FMI_10 : KIBES_Signal/KIBES_Signal  MBDS_LibraryBlock=on  DatabaseKey=158  SignalName=ICANDM1RxSA19.GenericDTCFilter.SPN_5_FMI_10  SymbolName=ICANDM1RxSA19_GenericDTCFilter_SPN_5_FMI_10_000158  DataType=boolean  Init=0  Slope=1  Bias=0  DataSize=1  fpDataType=boolean  BlockIOType=Inport  DeviceType=0
  in_ICANDM1RxSA19.GenericDTCFilter.SPN_6_FMI_1 : KIBES_Signal/KIBES_Signal  MBDS_LibraryBlock=on  DatabaseKey=159  SignalName=ICANDM1RxSA19.GenericDTCFilter.SPN_6_FMI_1  SymbolName=ICANDM1RxSA19_GenericDTCFilter_SPN_6_FMI_1_000159  DataType=boolean  Init=0  Slope=1  Bias=0  DataSize=1  fpDataType=boolean  BlockIOType=Inport  DeviceType=0
  in_IN_ICAN.IGenRx.I_Test1.MessageState : KIBES_Signal/KIBES_Signal  MBDS_LibraryBlock=on  DatabaseKey=90  SignalName=IN_ICAN.IGenRx.I_Test1.MessageState  SymbolName=IN_ICAN_IGenRx_I_Test1_MessageState_000090  DataType=uint16  Init=0  Slope=1  Bias=0  DataSize=1  fpDataType=uint16  BlockIOType=Inport  DeviceType=0
  in_IN_ICAN.IGenRx.I_Test1.Val_1 : KIBES_Signal/KIBES_Signal  MBDS_LibraryBlock=on  DatabaseKey=87  SignalName=IN_ICAN.IGenRx.I_Test1.Val_1  SymbolName=IN_ICAN_IGenRx_I_Test1_Val_1_000087  DataType=uint8  Init=0  Slope=1  Bias=0  DataSize=1  fpDataType=uint8  BlockIOType=Inport  DeviceType=0
  out_ICAN.ICANDM1RxSA19.MessageEnable : KIBES_Signal/KIBES_Signal  MBDS_LibraryBlock=on  DatabaseKey=154  SignalName=ICAN.ICANDM1RxSA19.MessageEnable  SymbolName=ICAN_ICANDM1RxSA19_MessageEnable_000154  DataType=boolean  Init=0  Slope=1  Bias=0  DataSize=1  fpDataType=boolean  BlockIOType=Outport  DeviceType=0
  out_ICAN.ICANDM1RxSAF1.MessageEnable : KIBES_Signal/KIBES_Signal  MBDS_LibraryBlock=on  DatabaseKey=138  SignalName=ICAN.ICANDM1RxSAF1.MessageEnable  SymbolName=ICAN_ICANDM1RxSAF1_MessageEnable_000138  DataType=boolean  Init=0  Slope=1  Bias=0  DataSize=1  fpDataType=boolean  BlockIOType=Outport  DeviceType=0
  out_ICAN.IPGNRX.PGRxMessage_1.Message_Enable : KIBES_Signal/KIBES_Signal  MBDS_LibraryBlock=on  DatabaseKey=452  SignalName=ICAN.IPGNRX.PGRxMessage_1.Message_Enable  SymbolName=ICAN_IPGNRX_PGRxMessage_1_Message_Enable_000452  DataType=boolean  Init=0  Slope=1  Bias=0  DataSize=1  fpDataType=boolean  BlockIOType=Outport  DeviceType=0
  out_OUT_ICAN.IGenRx.I_Test1.MessageEnable : KIBES_Signal/KIBES_Signal  MBDS_LibraryBlock=on  DatabaseKey=86  SignalName=OUT_ICAN.IGenRx.I_Test1.MessageEnable  SymbolName=OUT_ICAN_IGenRx_I_Test1_MessageEnable_000086  DataType=boolean  Init=0  Slope=1  Bias=0  DataSize=1  fpDataType=boolean  BlockIOType=Outport  DeviceType=0
  out_OUT_ICAN.IGenTx.I_Tes1.MessageEnable : KIBES_Signal/KIBES_Signal  MBDS_LibraryBlock=on  DatabaseKey=88  SignalName=OUT_ICAN.IGenTx.I_Tes1.MessageEnable  SymbolName=OUT_ICAN_IGenTx_I_Tes1_MessageEnable_000088  DataType=boolean  Init=0  Slope=1  Bias=0  DataSize=1  fpDataType=boolean  BlockIOType=Outport  DeviceType=0
  out_OUT_ICAN.IGenTx.I_Tes1.Val_1 : KIBES_Signal/KIBES_Signal  MBDS_LibraryBlock=on  DatabaseKey=89  SignalName=OUT_ICAN.IGenTx.I_Tes1.Val_1  SymbolName=OUT_ICAN_IGenTx_I_Tes1_Val_1_000089  DataType=uint8  Init=0  Slope=1  Bias=0  DataSize=1  fpDataType=uint8  BlockIOType=Outport  DeviceType=0
  wires:
  Constant8/1 -> out_ICAN.IPGNRX.PGRxMessage_1.Message_Enable/1
  Constant/1 -> out_ICAN.ICANDM1RxSA19.MessageEnable/1, out_ICAN.ICANDM1RxSAF1.MessageEnable/1, out_OUT_ICAN.IGenTx.I_Tes1.MessageEnable/1, out_OUT_ICAN.IGenRx.I_Test1.MessageEnable/1
  Constant3/1 -> out_OUT_ICAN.IGenTx.I_Tes1.Val_1/1

== system APP_MyApplication/Model/APP_MyApplication_/OR ==
  note: OR
  u1 : Inport  OutDataTypeStr=boolean
  u2 : Inport  Port=2  OutDataTypeStr=boolean
  u3 : Inport  Port=3  OutDataTypeStr=boolean
  u4 : Inport  Port=4  OutDataTypeStr=boolean
  DataType : DataTypeConversion  OutDataTypeStr=boolean
  Operator : Logic  Operator=OR  Inputs=4  AllPortsSameDT=off  OutDataTypeStr=boolean
  y : Outport
  wires:
  Operator/1 -> DataType/1
  u1/1 -> Operator/1
  u2/1 -> Operator/2
  DataType/1 -> y/1
  u3/1 -> Operator/3
  u4/1 -> Operator/4

== system APP_MyApplication/Model/APP_MyApplication_/Outputs ==
  Constant1 : Constant  InitFcn=|  Value=0  OutDataTypeStr=uint8
      | if(exist('MBDS_BlockCallback', 'file'))
      |    MBDS_BlockCallback('Update', gcb);  
      | end
  Constant8 : Constant  InitFcn=|  Value=0  OutDataTypeStr=uint8
      | if(exist('MBDS_BlockCallback', 'file'))
      |    MBDS_BlockCallback('Update', gcb);  
      | end
  Data Type Conversion : DataTypeConversion  InitFcn=|  SaturateOnIntegerOverflow=on
      | try
      |    MBDS_BlockCallback('Update', gcb);
      | end
      settings: AttributesFormatString=Saturate: %<SaturateOnIntegerOverflow>
  Switch : Switch  InitFcn=|  Criteria=u2 ~= 0  OutDataTypeStr=Inherit: Inherit via back propagation  mask(Switch){MBDS_LibraryBlock=on, OutDataTypeStr_=Inherit: Inherit via back propagation, SaturateOnIntegerOverflow_=off, InputSameDT_=off, MBDS_BlockVersion=07.21.05}
      | if(exist('MBDS_BlockCallback', 'file'))
      |    MBDS_BlockCallback('Update', gcb);  
      | end
      mask prompts: MBDS_LibraryBlock "MBDS library block"; OutDataTypeStr_ "Output data type:"; SaturateOnIntegerOverflow_ "Saturate on integer overflow"; InputSameDT_ "Require all inputs to have the same data type"; MBDS_BlockVersion "Block version:"
      mask help: Pass through input 1 when input 2 is not equal to zero; otherwise pass through input 3. The inputs are numbered top to bottom (or left to right). The first and third input ports are data ports, and the second input port is the control port.
      mask init: same as APP_MyApplication/Model/APP_MyApplication_/OR
      mask Help: eval(['open([workdir(''library_dir:''),''\Blockset\help\'',get_param(gcb,''MaskType''),''.html''])'])
      mask TypeOptions OutDataTypeStr_: Inherit: Inherit via back propagation | single | int8 | uint8 | int16 | uint16 | int32 | uint32
      mask DialogControl ParameterTabVar0 Prompt: Signal Attributes
      mask DialogControl ParameterTabVar01 Prompt: Version
  Switch1 : Switch  InitFcn=|  Criteria=u2 ~= 0  OutDataTypeStr=Inherit: Inherit via back propagation  mask(Switch){MBDS_LibraryBlock=on, OutDataTypeStr_=Inherit: Inherit via back propagation, SaturateOnIntegerOverflow_=off, InputSameDT_=off, MBDS_BlockVersion=07.21.05}
      | if(exist('MBDS_BlockCallback', 'file'))
      |    MBDS_BlockCallback('Update', gcb);  
      | end
      mask prompts: MBDS_LibraryBlock "MBDS library block"; OutDataTypeStr_ "Output data type:"; SaturateOnIntegerOverflow_ "Saturate on integer overflow"; InputSameDT_ "Require all inputs to have the same data type"; MBDS_BlockVersion "Block version:"
      mask help: Pass through input 1 when input 2 is not equal to zero; otherwise pass through input 3. The inputs are numbered top to bottom (or left to right). The first and third input ports are data ports, and the second input port is the control port.
      mask init: same as APP_MyApplication/Model/APP_MyApplication_/OR
      mask Help: eval(['open([workdir(''library_dir:''),''\Blockset\help\'',get_param(gcb,''MaskType''),''.html''])'])
      mask TypeOptions OutDataTypeStr_: Inherit: Inherit via back propagation | single | int8 | uint8 | int16 | uint16 | int32 | uint32
      mask DialogControl ParameterTabVar0 Prompt: Signal Attributes
      mask DialogControl ParameterTabVar01 Prompt: Version
  in_DIAG_DigitalOutputsSTATIC.OUT_01_DIAG : KIBES_Signal/KIBES_Signal  MBDS_LibraryBlock=on  DatabaseKey=82  SignalName=DIAG_DigitalOutputsSTATIC.OUT_01_DIAG  SymbolName=DIAG_DigitalOutputsSTATIC_OUT_01_DIAG_000082  DataType=uint16  Init=1  Slope=1  Bias=0  DataSize=1  fpDataType=uint16  BlockIOType=Inport  DeviceType=0
  in_DigitalOutputPWM.OUT_20_PWM_DIAG : KIBES_Signal/KIBES_Signal  MBDS_LibraryBlock=on  DatabaseKey=221  SignalName=DigitalOutputPWM.OUT_20_PWM_DIAG  SymbolName=DigitalOutputPWM_OUT_20_PWM_DIAG_000221  DataType=uint16  Init=1  Slope=1  Bias=0  DataSize=1  fpDataType=uint16  BlockIOType=Inport  DeviceType=0
  in_DigitalOutputPWM.OUT_20_TD : KIBES_Signal/KIBES_Signal  MBDS_LibraryBlock=on  DatabaseKey=222  SignalName=DigitalOutputPWM.OUT_20_TD  SymbolName=DigitalOutputPWM_OUT_20_TD_000222  DataType=boolean  Init=0  Slope=1  Bias=0  DataSize=1  fpDataType=boolean  BlockIOType=Inport  DeviceType=0
  in_DigitalOutputPWM.OUT_20_TD_DIAG : KIBES_Signal/KIBES_Signal  MBDS_LibraryBlock=on  DatabaseKey=223  SignalName=DigitalOutputPWM.OUT_20_TD_DIAG  SymbolName=DigitalOutputPWM_OUT_20_TD_DIAG_000223  DataType=uint16  Init=1  Slope=1  Bias=0  DataSize=1  fpDataType=uint16  BlockIOType=Inport  DeviceType=0
  in_DigitalOutputsSTATIC.OUT_01_TD : KIBES_Signal/KIBES_Signal  MBDS_LibraryBlock=on  DatabaseKey=217  SignalName=DigitalOutputsSTATIC.OUT_01_TD  SymbolName=DigitalOutputsSTATIC_OUT_01_TD_000217  DataType=boolean  Init=0  Slope=1  Bias=0  DataSize=1  fpDataType=boolean  BlockIOType=Inport  DeviceType=0
  in_DigitalOutputsSTATIC.OUT_01_TD_DIAG : KIBES_Signal/KIBES_Signal  MBDS_LibraryBlock=on  DatabaseKey=263  SignalName=DigitalOutputsSTATIC.OUT_01_TD_DIAG  SymbolName=DigitalOutputsSTATIC_OUT_01_TD_DIAG_000263  DataType=uint16  Init=1  Slope=1  Bias=0  DataSize=1  fpDataType=uint16  BlockIOType=Inport  DeviceType=0
  in_DigitalOutputsSTATIC.OUT_04_DIAG : KIBES_Signal/KIBES_Signal  MBDS_LibraryBlock=on  DatabaseKey=229  SignalName=DigitalOutputsSTATIC.OUT_04_DIAG  SymbolName=DigitalOutputsSTATIC_OUT_04_DIAG_000229  DataType=uint16  Init=1  Slope=1  Bias=0  DataSize=1  fpDataType=uint16  BlockIOType=Inport  DeviceType=0
  in_DigitalOutputsSTATIC.OUT_04_TD : KIBES_Signal/KIBES_Signal  MBDS_LibraryBlock=on  DatabaseKey=230  SignalName=DigitalOutputsSTATIC.OUT_04_TD  SymbolName=DigitalOutputsSTATIC_OUT_04_TD_000230  DataType=boolean  Init=0  Slope=1  Bias=0  DataSize=1  fpDataType=boolean  BlockIOType=Inport  DeviceType=0
  in_DigitalOutputsSTATIC.OUT_04_TD_DIAG : KIBES_Signal/KIBES_Signal  MBDS_LibraryBlock=on  DatabaseKey=231  SignalName=DigitalOutputsSTATIC.OUT_04_TD_DIAG  SymbolName=DigitalOutputsSTATIC_OUT_04_TD_DIAG_000231  DataType=uint16  Init=1  Slope=1  Bias=0  DataSize=1  fpDataType=uint16  BlockIOType=Inport  DeviceType=0
  in_STIMD.OUT_TdActivation : KIBES_Signal/KIBES_Signal  MBDS_LibraryBlock=on  DatabaseKey=225  SignalName=STIMD.OUT_TdActivation  SymbolName=STIMD_OUT_TdActivation_000225  DataType=boolean  Init=0  Slope=1  Bias=0  DataSize=1  fpDataType=boolean  BlockIOType=Inport  DeviceType=2
  in_STIMD.OUT_enable : KIBES_Signal/KIBES_Signal  MBDS_LibraryBlock=on  DatabaseKey=227  SignalName=STIMD.OUT_enable  SymbolName=STIMD_OUT_enable_000227  DataType=boolean  Init=0  Slope=1  Bias=0  DataSize=1  fpDataType=boolean  BlockIOType=Inport  DeviceType=2
  in_STIMD.OUT_value : KIBES_Signal/KIBES_Signal  MBDS_LibraryBlock=on  DatabaseKey=226  SignalName=STIMD.OUT_value  SymbolName=STIMD_OUT_value_000226  DataType=uint8  Init=0  Slope=1  Bias=0  DataSize=1  fpDataType=uint8  BlockIOType=Inport  DeviceType=2
  out_DigitalOutputPWM.OUT_20_PWM : KIBES_Signal/KIBES_Signal  MBDS_LibraryBlock=on  DatabaseKey=220  SignalName=DigitalOutputPWM.OUT_20_PWM  SymbolName=DigitalOutputPWM_OUT_20_PWM_000220  DataType=uint8  Init=0  Slope=1  Bias=0  DataSize=1  fpDataType=uint8  BlockIOType=Outport  DeviceType=0
  out_DigitalOutputPWM.OUT_20_TD_START : KIBES_Signal/KIBES_Signal  MBDS_LibraryBlock=on  DatabaseKey=224  SignalName=DigitalOutputPWM.OUT_20_TD_START  SymbolName=DigitalOutputPWM_OUT_20_TD_START_000224  DataType=boolean  Init=0  Slope=1  Bias=0  DataSize=1  fpDataType=boolean  BlockIOType=Outport  DeviceType=0
  out_DigitalOutputsSTATIC.OUT_01_TD_START : KIBES_Signal/KIBES_Signal  MBDS_LibraryBlock=on  DatabaseKey=219  SignalName=DigitalOutputsSTATIC.OUT_01_TD_START  SymbolName=DigitalOutputsSTATIC_OUT_01_TD_START_000219  DataType=boolean  Init=0  Slope=1  Bias=0  DataSize=1  fpDataType=boolean  BlockIOType=Outport  DeviceType=0
  out_DigitalOutputsSTATIC.OUT_04 : KIBES_Signal/KIBES_Signal  MBDS_LibraryBlock=on  DatabaseKey=228  SignalName=DigitalOutputsSTATIC.OUT_04  SymbolName=DigitalOutputsSTATIC_OUT_04_000228  DataType=boolean  Init=0  Slope=1  Bias=0  DataSize=1  fpDataType=boolean  BlockIOType=Outport  DeviceType=0
  out_DigitalOutputsSTATIC.OUT_04_TD_START : KIBES_Signal/KIBES_Signal  MBDS_LibraryBlock=on  DatabaseKey=232  SignalName=DigitalOutputsSTATIC.OUT_04_TD_START  SymbolName=DigitalOutputsSTATIC_OUT_04_TD_START_000232  DataType=boolean  Init=0  Slope=1  Bias=0  DataSize=1  fpDataType=boolean  BlockIOType=Outport  DeviceType=0
  out_OUT_DigitalOutputsSTATIC.OUT_01 : KIBES_Signal/KIBES_Signal  MBDS_LibraryBlock=on  DatabaseKey=81  SignalName=OUT_DigitalOutputsSTATIC.OUT_01  SymbolName=OUT_DigitalOutputsSTATIC_OUT_01_000081  DataType=boolean  Init=0  Slope=1  Bias=0  DataSize=1  fpDataType=boolean  BlockIOType=Outport  DeviceType=0
  wires:
  in_STIMD.OUT_enable/1 -> Switch1/2, Switch/2
  Constant8/1 -> Switch/3
  in_STIMD.OUT_value/1 -> Switch/1
  Switch/1 -> out_DigitalOutputPWM.OUT_20_PWM/1, Data Type Conversion/1
  Constant1/1 -> Switch1/3
  in_STIMD.OUT_TdActivation/1 -> Switch1/1
  Switch1/1 -> out_DigitalOutputsSTATIC.OUT_04_TD_START/1, out_DigitalOutputPWM.OUT_20_TD_START/1, out_DigitalOutputsSTATIC.OUT_01_TD_START/1
  Data Type Conversion/1 -> out_DigitalOutputsSTATIC.OUT_04/1, out_OUT_DigitalOutputsSTATIC.OUT_01/1
